simulink model "model_eq_wfa"  (R2020b)
settings: Solver=VariableStepAuto  StartTime=0.0  StopTime=1  RelTol=1e-3
values from neighbouring files (symbols this model uses):
  in_cos = 2*cos(2*pi*k/N)    [compute_constants.m]    (also in signat_to_test_generate.m = -2*cos(2*pi*k/N))
  Wkn = -exp(-j*2*pi*k/N)    [compute_constants.m]    (also in signat_to_test_generate.m)
undefined symbols (not defined in the file or in its folder): dfilt
libraries: simulink x2, dsparch4 x1
settings Model: Creator=pablo  LastModifiedBy=pablo

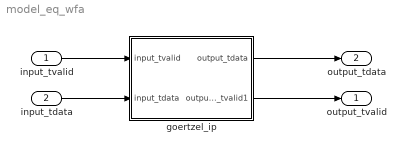
== system model_eq_wfa ==
  input_tvalid : Inport
  input_tdata : Inport  Port=2
  goertzel_ip : Subsystem
  output_tvalid : Outport
  output_tdata : Outport  Port=2
  wires:
  goertzel_ip/1(output_tdata) -> output_tdata/1
  input_tvalid/1 -> goertzel_ip/1(input_tvalid)
  input_tdata/1 -> goertzel_ip/2(input_tdata)
  goertzel_ip/2(output_tvalid1) -> output_tvalid/1

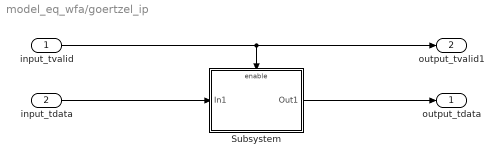
== system model_eq_wfa/goertzel_ip ==
  input_tvalid : Inport  OutDataTypeStr=boolean
  input_tdata : Inport  Port=2
  Subsystem : Subsystem
  output_tdata : Outport
  output_tvalid1 : Outport  Port=2  InitialOutput=0
  wires:
  input_tdata/1 -> Subsystem/1(In1)
  Subsystem/1(Out1) -> output_tdata/1
  input_tvalid/1 -> output_tvalid1/1, Subsystem/Enable

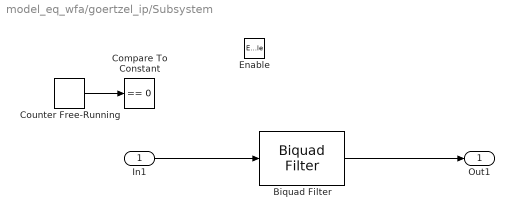
== system model_eq_wfa/goertzel_ip/Subsystem ==
  In1 : Inport  OutDataTypeStr=fixdt(1,32,16)
  Enable : EnablePort
  Biquad Filter : dsparch4/Biquad Filter  FilterSource=Dialog parameters  CoeffSource=Specify via dialog  FilterObject=dfilt.df2tsos([1 0.3 0.4],[1 0.1 0.2])  IIRFiltStruct=Direct form II transposed  BiQuadCoeffs=[0 1 real(Wkn) 1 -in_cos 1]  ScaleValues=1  IC=0  ICnum=0  ICden=0  a0Flag=Warning  optimizeScaleValues=on  ScaleValueMode=Specify via input port (g)  roundingMode=Floor  overflowMode=off  scaleValueFracLength=14  denProdOutputFracLength=30  denAccumFracLength=30  secondMemoryFracLength=15
      settings: SourceProductName=DSP System Toolbox
  Compare To Constant : simulink/Logic and Bit Operations/Compare To Constant  relop===  const=0  OutDataTypeStr=boolean
  Counter Free-Running : simulink/Sources/Counter Free-Running  NumBits=5  tsamp=-1
  Out1 : Outport  InitialOutput=0
  wires:
  Biquad Filter/1 -> Out1/1
  In1/1 -> Biquad Filter/1
  Counter Free-Running/1 -> Compare To Constant/1
